simulink model "template_drone"  (R2020b)
settings: Solver=FixedStepAuto  StartTime=0.0  StopTime=100  RelTol=1e-3  EnableMultiTasking=on
InitFcn:
  | load('BusDefinitions.mat')
  | codertarget.parrot.internal.checkImageBlocks(gcs)
undefined symbols (not defined in the file): codertarget, enableLanding, Estimator, landingAltitude, Rec, SDTV, Ts
libraries: visionconversions x11, visionstatistics x10, simulink x7, parrotlib x1
(part 2 of 2)

== matlab function template_drone/Flight Control System/controller_new/Waypoint_switcher/MATLAB Function ==
  data: pos input; cwp output double size=[3]; yaw output double; travel_dist input; action input; old_yaw input; cwp_old input
function [cwp, yaw] = waypoint_switcher(pos, travel_dist, action, old_yaw, cwp_old)

travel_dist = 2

Radius = 0.2

cwp = cwp_old
waypoint_yaw = old_yaw

if in_range(pos(1), cwp(1), pos(2), cwp(2), pos(3), cwp(3), Radius) ==1
        move = 1
        
        switch action
            case 1
                waypoint_yaw = waypoint_yaw + 1.57
            case 2
                waypoint_yaw = waypoint_yaw- 1.57
            case 3
                waypoint_yaw = waypoint_yaw
            otherwise
                move = 0
        end
              
        if move == 1
            dir = get_direction(waypoint_yaw)*travel_dist
            cwp(1) = cwp(1)+dir(1)
            cwp(2) = cwp(2)+dir(2)
        end
    
end
    
cwp = cwp
yaw =  waypoint_yaw

end

function bool = in_range(x_a, x_b, y_a, y_b, z_a, z_b, Radius)
    bool = 0;
    range = sqrt( (x_a-x_b)^2 + (y_a-y_b)^2 + (z_a-z_b)^2);
    if range <= Radius
        bool = 1;             
    end
end

function direction_vec = get_direction(waypoint_yaw)
    waypoint_x = cos(waypoint_yaw) 
    waypoint_y = sin(waypoint_yaw)
    direction_vec = [waypoint_x waypoint_y]
end

== matlab function template_drone/Image Processing System/colour_detect/MATLAB Function ==
  data: red_count input; action output; blue_count input; green_count input; purple_count input
function action = fcn(red_count, blue_count, green_count, purple_count)
    
%     switch colour
%         case red_count >= 1
%             action = 1; %% turns left
%         case blue_count >= 1
%             action = 2; %% turns right
%         case green_count >= 1
%             action = 3; %% flies forward
%         case purple_count >=1
%             action = 4; %% flies backwards
%         otherwise
%             action = 0; %% dont do anything/ fly forward 
%     end
    if red_count >= 1
        action = 1;
            else
        action = 0;
    end
    if blue_count >= 1
        action = 2;
    end
    if green_count >= 1
        action = 3;
    end
    if purple_count >= 1
        action  =4;
    end
    
    action = 1;
end

== matlab function template_drone/Image Processing System/colour_detect/MATLAB Function1 ==
  data: r input; y output; g input; b input
function y = fcn(r, g, b)



y = u;

== matlab function template_drone/Image Processing System/colour_detect/MATLAB Function2 ==
  data: r input; action output; g input; b input
function action = fcn(r, g, b)
    low = 400;
    high = 2000;
    
    red = threshold(r, low, high);
    green = threshold(g, low, high);
    blue = threshold(b, low, high);
    
    [M, action] = max([0 red*r green*g blue*b]);
    action = action - 1;
    
end

function bool = threshold(num, low, high)
    if num > low
        if high > num
            bool = 1;
        else 
            bool = 0;
        end
    else 
        bool = 0;
    end
end

== matlab function template_drone/Image Processing System/colour_detect/MATLAB Function3 ==
  data: r input; BW output; g input; b input; desired_color input; threshold input
function BW = color_mask(r, g, b, desired_color, threshold)
    [x, y] = size(r);
    BW = zeros(x, y);
    for i = 1:x
        for j = 1:y
%             color_tested = double([r(i, j), g(i, j), b(i, j)])
%             desired_col = double(desired_color')
%             subtract = color_tested - desired_col
            dist = distance(double([r(i, j), g(i, j), b(i, j)]), double(desired_color'));
            if dist > threshold
                BW(i, j) = 1;
            end
        end
    end   
end

function d = distance(col_a, col_b)
    d = abs(norm(col_a-col_b));
    %new= sqrt(matrix1.^2+matrix2.^2)

end

== matlab function template_drone/Image Processing System/MATLAB Function2 ==
  data: r input; action output; g input; b input
function action = fcn(r, g, b)
    low = 400;
    high = 2000;
    
    red = threshold(r, low, high);
    green = threshold(g, low, high);
    blue = threshold(b, low, high);
    
    [M, action] = max([0 red*r green*g blue*b])
    action = action - 1
    
end

function bool = threshold(num, low, high)
    if num > low
        if high > num
            bool = 1;
        else 
            bool = 0;
        end
    else 
        bool = 0;
    end
end
